simulink model "inversor"  (R2018a)
settings: Solver=VariableStepAuto  StartTime=0.0  StopTime=2  MaxStep=1e-4  RelTol=1e-3
InitFcn:
  | stateStadeInv
  | MODELOHIDROV8
undefined symbols (not defined in the file): Fr, sigbuilder_block
libraries: simulink x2, powerlib x1
settings Model: Creator=Hp 14  LastModifiedBy=cmparedes

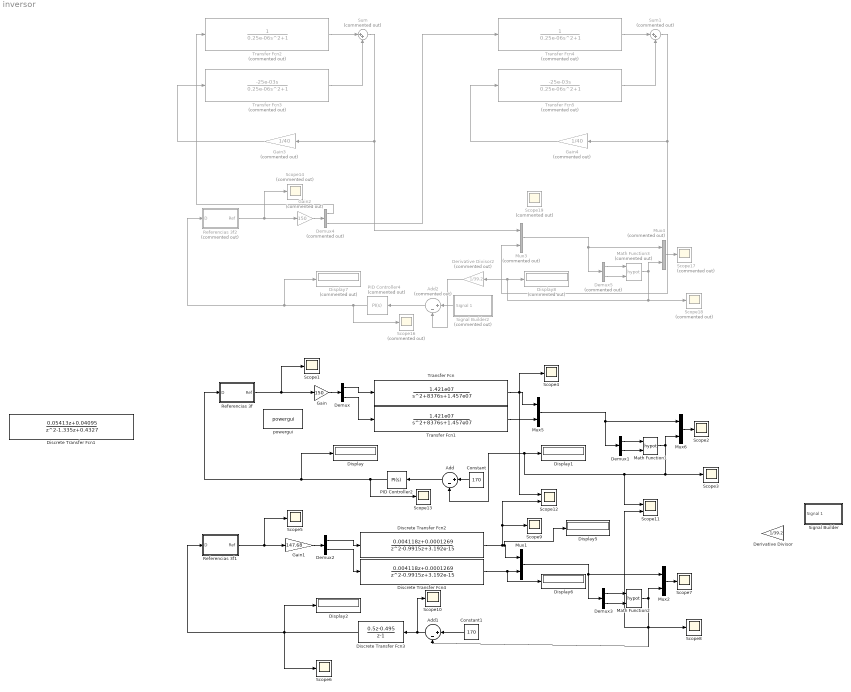
== system inversor ==
  Add : Sum  Inputs=|+-
  Add1 : Sum  Inputs=|+-
  Add2 : Sum  Commented=on  Inputs=|+-
  Constant : Constant  Value=170
  Constant1 : Constant  Value=170
  Demux{,1..3} (4 alike) : Demux  Outputs=2
  Demux4 : Demux  Commented=on  Outputs=2
  Demux5 : Demux  Commented=on  Outputs=2
  Derivative Divisor : Gain  Gain=1/39.2  SaturateOnIntegerOverflow=on  OutDataTypeStr=Inherit: Same as input  ParamDataTypeStr=Inherit: Same as input
  Derivative Divisor2 : Gain  Commented=on  Gain=1/39.2  SaturateOnIntegerOverflow=on  OutDataTypeStr=Inherit: Same as input  ParamDataTypeStr=Inherit: Same as input
  Discrete Transfer Fcn1 : DiscreteTransferFcn  Numerator=[0.05413 0.04095]  Denominator=[1 -1.335 0.4327]
  Discrete Transfer Fcn2 : DiscreteTransferFcn  Numerator=[0.004118 0.0001269]  Denominator=[1 -0.9915 3.192e-15]
  Discrete Transfer Fcn3 : DiscreteTransferFcn  Numerator=[0.5 -0.495]  Denominator=[1 -1]
  Discrete Transfer Fcn4 : DiscreteTransferFcn  Numerator=[0.004118 0.0001269]  Denominator=[1 -0.9915 3.192e-15]
  Display{,1..2,5..6} (5 alike) : Display
  Display7 : Display  Commented=on
  Display8 : Display  Commented=on
  Gain : Gain  Gain=150
  Gain1 : Gain  Gain=147.68
  Gain2 : Gain  Commented=on  Gain=150
  Gain3 : Gain  Commented=on  Gain=1/40
  Gain4 : Gain  Commented=on  Gain=1/40
  Math Function1 : Math  Operator=hypot  SaturateOnIntegerOverflow=on
  Math Function2 : Math  Operator=hypot  SaturateOnIntegerOverflow=on
  Math Function3 : Math  Commented=on  Operator=hypot  SaturateOnIntegerOverflow=on
  Mux{1..2,5..6} (4 alike) : Mux  Inputs=2
  Mux3 : Mux  Commented=on  Inputs=2
  Mux4 : Mux  Commented=on  Inputs=2
  PID Controller2 : simulink/Continuous/PID Controller  Controller=PI  TimeDomain=Continuous-time  SampleTime=-1  IntegratorMethod=Forward Euler  FilterMethod=Forward Euler  Form=Parallel  UseFilter=on  ControllerParametersSource=internal  P=0.5  I=50  D=0  N=100  InitialConditionSource=internal  InitialConditionForIntegrator=0  InitialConditionForFilter=0  ExternalReset=none  LimitOutput=off  UpperSaturationLimit=inf  LowerSaturationLimit=-inf  LinearizeAsGain=on  AntiWindupMode=none  Kb=1  TrackingMode=off  Kt=1  PParamMin=[]  PParamMax=[]  IParamMin=[]  IParamMax=[]  DParamMin=[]  DParamMax=[]  NParamMin=[]  NParamMax=[]  KbParamMin=[]  KbParamMax=[]  KtParamMin=[]  KtParamMax=[]  POutMin=[]  POutMax=[]  IOutMin=[]  IOutMax=[]  DOutMin=[]  DOutMax=[]  NOutMin=[]  NOutMax=[]  KbOutMin=[]  KbOutMax=[]  KtOutMin=[]  KtOutMax=[]  IntegratorOutMin=[]  IntegratorOutMax=[]  FilterOutMin=[]  FilterOutMax=[]  SumOutMin=[]  SumOutMax=[]  SumI1OutMin=[]  SumI1OutMax=[]  SumI2OutMin=[]  SumI2OutMax=[]  SumI3OutMin=[]  SumI3OutMax=[]  SumDOutMin=[]  SumDOutMax=[]  SaturationOutMin=[]  SaturationOutMax=[]  IntegratorContinuousStateAttributes=''  IntegratorStateMustResolveToSignalObject=off  IntegratorRTWStateStorageClass=Auto  FilterContinuousStateAttributes=''  FilterStateMustResolveToSignalObject=off  FilterRTWStateStorageClass=Auto  DifferentiatorICPrevScaledInput=0  DifferentiatorOutMin=[]  DifferentiatorOutMax=[]  InitialConditionSetting=State (most efficient)  FilterDiffOutCoefMin=[]  FilterDiffOutCoefMax=[]  SumDenOutMin=[]  SumDenOutMax=[]  SumNumOutMin=[]  SumNumOutMax=[]  ReciprocalOutMin=[]  ReciprocalOutMax=[]  DivideOutMin=[]  DivideOutMax=[]  TunerSelectOption=Transfer Function Based (PID Tuner App)
  PID Controller4 : simulink/Continuous/PID Controller  Commented=on  Controller=PI  TimeDomain=Continuous-time  SampleTime=-1  IntegratorMethod=Forward Euler  FilterMethod=Forward Euler  Form=Parallel  UseFilter=on  ControllerParametersSource=internal  P=0.5  I=50  D=0  N=100  InitialConditionSource=internal  InitialConditionForIntegrator=0  InitialConditionForFilter=0  ExternalReset=none  LimitOutput=off  UpperSaturationLimit=inf  LowerSaturationLimit=-inf  LinearizeAsGain=on  AntiWindupMode=none  Kb=1  TrackingMode=off  Kt=1  PParamMin=[]  PParamMax=[]  IParamMin=[]  IParamMax=[]  DParamMin=[]  DParamMax=[]  NParamMin=[]  NParamMax=[]  KbParamMin=[]  KbParamMax=[]  KtParamMin=[]  KtParamMax=[]  POutMin=[]  POutMax=[]  IOutMin=[]  IOutMax=[]  DOutMin=[]  DOutMax=[]  NOutMin=[]  NOutMax=[]  KbOutMin=[]  KbOutMax=[]  KtOutMin=[]  KtOutMax=[]  IntegratorOutMin=[]  IntegratorOutMax=[]  FilterOutMin=[]  FilterOutMax=[]  SumOutMin=[]  SumOutMax=[]  SumI1OutMin=[]  SumI1OutMax=[]  SumI2OutMin=[]  SumI2OutMax=[]  SumI3OutMin=[]  SumI3OutMax=[]  SumDOutMin=[]  SumDOutMax=[]  SaturationOutMin=[]  SaturationOutMax=[]  IntegratorContinuousStateAttributes=''  IntegratorStateMustResolveToSignalObject=off  IntegratorRTWStateStorageClass=Auto  FilterContinuousStateAttributes=''  FilterStateMustResolveToSignalObject=off  FilterRTWStateStorageClass=Auto  DifferentiatorICPrevScaledInput=0  DifferentiatorOutMin=[]  DifferentiatorOutMax=[]  InitialConditionSetting=State (most efficient)  FilterDiffOutCoefMin=[]  FilterDiffOutCoefMax=[]  SumDenOutMin=[]  SumDenOutMax=[]  SumNumOutMin=[]  SumNumOutMax=[]  ReciprocalOutMin=[]  ReciprocalOutMax=[]  DivideOutMin=[]  DivideOutMax=[]  TunerSelectOption=Transfer Function Based (PID Tuner App)
  Referencias 3f : Subsystem
  Referencias 3f1 : Subsystem
  Referencias 3f2 : Subsystem  Commented=on
  Scope{1..10,13} (11 alike) : Scope
  Scope11 : Scope  NumInputPorts=2
  Scope12 : Scope  NumInputPorts=2
  Scope{14,16..19} (5 alike) : Scope  Commented=on
  Signal Builder : Subsystem  Tag=STV Subsys  LoadFcn=sigbuilder_block('load');  StartFcn=sigbuilder_block('start');  StopFcn=sigbuilder_block('stop');  ClipboardFcn=sigbuilder_block('clipboard');  mask(Sigbuilder block){tuvar=[0:10]}
      mask help: Sigbuilder GUI
      mask init:
      | if ~strcmp(get_param(bdroot(gcbh),'SimulationStatus'),'stopped') tuvar = sigbuilder_block('maskInit'); end
      settings: CopyFcn=sigbuilder_block('copy');  DeleteFcn=sigbuilder_block('delete');  ModelCloseFcn=sigbuilder_block('modelClose');  PreSaveFcn=sigbuilder_block('preSave');  PauseFcn=sigbuilder_block('pause')  ContinueFcn=sigbuilder_block('continue')  NameChangeFcn=sigbuilder_block('namechange');  OpenFcn=sigbuilder_block('open',[6 24 765 492 ]);  CloseFcn=sigbuilder_block('close');
      mask Display: plot(0, 0, 100, 100,[2, 2, 32, 32, 2], [68, 8, 8, 68, 68],[32, 2], [38, 38], [32, 19, 2],[53, 60, 44], [32, 17, 17, 2],[16, 16, 31, 31]);txt = getActiveGroup(gcbh);text(2, 100, txt,'verticalAlignment', 'top');
  Signal Builder2 : Subsystem  Tag=STV Subsys  Commented=on  LoadFcn=sigbuilder_block('load');  StartFcn=sigbuilder_block('start');  StopFcn=sigbuilder_block('stop');  ClipboardFcn=sigbuilder_block('clipboard');  mask(Sigbuilder block){tuvar=[0:10]}
      mask help: Sigbuilder GUI
      mask init:
      | if ~strcmp(get_param(bdroot(gcbh),'SimulationStatus'),'stopped') tuvar = sigbuilder_block('maskInit'); end
      settings: CopyFcn=sigbuilder_block('copy');  DeleteFcn=sigbuilder_block('delete');  ModelCloseFcn=sigbuilder_block('modelClose');  PreSaveFcn=sigbuilder_block('preSave');  PauseFcn=sigbuilder_block('pause')  ContinueFcn=sigbuilder_block('continue')  NameChangeFcn=sigbuilder_block('namechange');  OpenFcn=sigbuilder_block('open',[6 24 765 492 ]);  CloseFcn=sigbuilder_block('close');
      mask Display: plot(0, 0, 100, 100,[2, 2, 32, 32, 2], [68, 8, 8, 68, 68],[32, 2], [38, 38], [32, 19, 2],[53, 60, 44], [32, 17, 17, 2],[16, 16, 31, 31]);txt = getActiveGroup(gcbh);text(2, 100, txt,'verticalAlignment', 'top');
  Sum : Sum  Commented=on  Inputs=|++
  Sum1 : Sum  Commented=on  Inputs=|++
  Transfer Fcn : TransferFcn  Numerator=[1.421e07]  Denominator=[1 8376 1.457e07]
  Transfer Fcn1 : TransferFcn  Numerator=[1.421e07]  Denominator=[1 8376 1.457e07]
  Transfer Fcn2 : TransferFcn  Commented=on  Denominator=[0.25e-06 0 1]
  Transfer Fcn3 : TransferFcn  Commented=on  Numerator=[-25e-03 0]  Denominator=[0.25e-06 0 1]
  Transfer Fcn4 : TransferFcn  Commented=on  Denominator=[0.25e-06 0 1]
  Transfer Fcn5 : TransferFcn  Commented=on  Numerator=[-25e-03 0]  Denominator=[0.25e-06 0 1]
  powergui : powerlib/powergui  Priority=1  SimulationMode=Continuous  SampleTime=50e-3  frequency=60  Iterations=50  frequencyindice=0  Pbase=100e6  ErrMax=1e-4  UnitsV=kV  UnitsW=MW  buscounter=0  FunctionMessages=off  echomessages=off  EnableUseOfTLC=off  CurrentSourceSwitches=off  DisableSnubberDevices=off  DisableRonSwitches=off  DisableVfSwitches=off  DisplayEquations=off  SolverType=Tustin/Backward Euler (TBE)  Interpol=off  ExternalGateDelay=off  methode=off  Ts=100  x0status=blocks  SPID=on  SwTol=0  HookPort=off  RestoreLinks=warning  ResistiveCurrentMeasurement=off  Frange=[0:2:500]  Ylog=off  Xlog=on  ShowGrid=off  save=off  variable=ZData  structure=0  ZoomFFT=off  StartTime=0.0  cycles=1  DisplayStyle=1  fundamental=60  FreqAxis=off  MaxFrequency=1000  frequencyindicesteady=0 Hz  RmsSteady=1  display=off
  wires:
  Transfer Fcn1/1 -> Mux5/2
  Transfer Fcn/1 -> Scope12/1, Scope4/1, Mux5/1
  Demux1/1 -> Math Function1/1
  Mux5/1 -> Demux1/1, Mux6/1
  Mux6/1 -> Scope2/1
  Demux1/2 -> Math Function1/2
  Referencias 3f/1(Ref) -> Gain/1, Scope1/1
  Demux/1 -> Transfer Fcn/1
  Demux/2 -> Transfer Fcn1/1
  Gain/1 -> Demux/1
  PID Controller2/1 -> Display/1, Referencias 3f/1(D), Scope13/1
  Constant/1 -> Add/1
  Add/1 -> PID Controller2/1
  Math Function1/1 -> Mux6/2, Scope3/1, Add/2, Display1/1, Scope11/1
  Add1/1 -> Discrete Transfer Fcn3/1, Scope10/1
  Math Function2/1 -> Add1/2, Scope11/2, Scope8/1, Mux2/2
  Discrete Transfer Fcn3/1 -> Scope6/1, Referencias 3f1/1(D), Display2/1
  Referencias 3f1/1(Ref) -> Scope5/1, Gain1/1
  Demux3/2 -> Math Function2/2
  Mux2/1 -> Scope7/1
  Mux1/1 -> Mux2/1, Demux3/1
  Demux3/1 -> Math Function2/1
  Discrete Transfer Fcn2/1 -> Display5/1, Mux1/1, Scope12/2, Scope9/1
  Discrete Transfer Fcn4/1 -> Display6/1, Mux1/2
  Gain1/1 -> Demux2/1
  Demux2/1 -> Discrete Transfer Fcn2/1
  Demux2/2 -> Discrete Transfer Fcn4/1
  Derivative Divisor2/1 -> Add2/2
  Add2/1 -> PID Controller4/1
  Math Function3/1 -> Display8/1, Derivative Divisor2/1, Scope18/1, Mux4/2
  Signal Builder2/1(Signal 1) -> Add2/1
  PID Controller4/1 -> Scope16/1, Referencias 3f2/1(D), Display7/1
  Gain2/1 -> Demux4/1
  Referencias 3f2/1(Ref) -> Scope14/1, Gain2/1
  Demux5/2 -> Math Function3/2
  Mux4/1 -> Scope17/1
  Mux3/1 -> Mux4/1, Demux5/1
  Demux5/1 -> Math Function3/1
  Demux4/1 -> Transfer Fcn2/1
  Gain3/1 -> Transfer Fcn3/1
  Transfer Fcn2/1 -> Sum/1
  Sum/1 -> Mux3/1, Gain3/1
  Transfer Fcn3/1 -> Sum/2
  Transfer Fcn5/1 -> Sum1/2
  Sum1/1 -> Mux3/2, Gain4/1
  Transfer Fcn4/1 -> Sum1/1
  Gain4/1 -> Transfer Fcn5/1
  Demux4/2 -> Transfer Fcn4/1
  Constant1/1 -> Add1/1

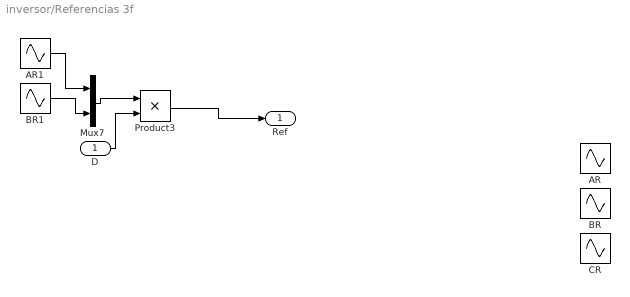
== system inversor/Referencias 3f ==
  D : Inport
  AR : Sin  Frequency=Fr*2*pi  SampleTime=0
  AR1 : Sin  Frequency=Fr*2*pi  SampleTime=0
  BR : Sin  Frequency=Fr*2*pi  Phase=-2*pi/3  SampleTime=0
  BR1 : Sin  Frequency=Fr*2*pi  Phase=-pi/2  SampleTime=0
  CR : Sin  Frequency=Fr*2*pi  Phase=2*pi/3  SampleTime=0
  Mux7 : Mux  Inputs=2
  Product3 : Product  OutDataTypeStr=double  RndMeth=Zero
  Ref : Outport
  wires:
  BR1/1 -> Mux7/2
  AR1/1 -> Mux7/1
  Mux7/1 -> Product3/1
  D/1 -> Product3/2
  Product3/1 -> Ref/1

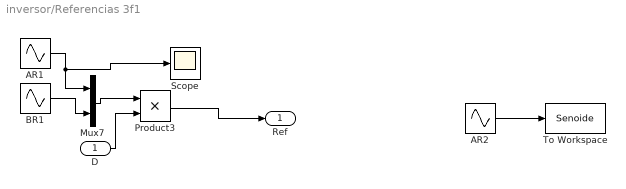
== system inversor/Referencias 3f1 ==
  D : Inport
  AR1 : Sin  Frequency=Fr*2*pi  SampleTime=0
  AR2 : Sin  Frequency=Fr*2*pi  SampleTime=0
  BR1 : Sin  Frequency=Fr*2*pi  Phase=-pi/2  SampleTime=0
  Mux7 : Mux  Inputs=2
  Product3 : Product  OutDataTypeStr=double  RndMeth=Zero
  Scope : Scope
  To Workspace : ToWorkspace  VariableName=Senoide  SaveFormat=Timeseries  SampleTime=-1
  Ref : Outport
  wires:
  Product3/1 -> Ref/1
  D/1 -> Product3/2
  Mux7/1 -> Product3/1
  AR1/1 -> Scope/1, Mux7/1
  BR1/1 -> Mux7/2
  AR2/1 -> To Workspace/1

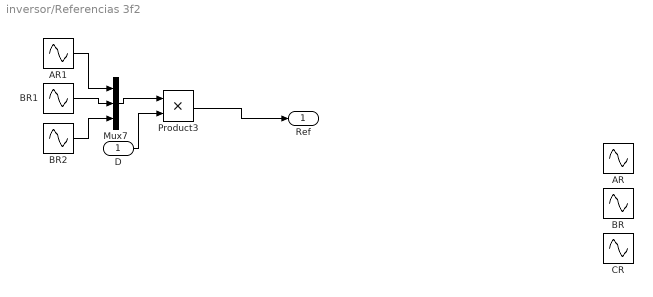
== system inversor/Referencias 3f2 ==
  D : Inport
  AR : Sin  Frequency=Fr*2*pi  SampleTime=0
  AR1 : Sin  Frequency=Fr*2*pi  SampleTime=0
  BR : Sin  Frequency=Fr*2*pi  Phase=-2*pi/3  SampleTime=0
  BR1 : Sin  Frequency=Fr*2*pi  Phase=-pi/2  SampleTime=0
  BR2 : Sin  Frequency=Fr*2*pi  Phase=pi/2  SampleTime=0
  CR : Sin  Frequency=Fr*2*pi  Phase=2*pi/3  SampleTime=0
  Mux7 : Mux  Inputs=3
  Product3 : Product  OutDataTypeStr=double  RndMeth=Zero
  Ref : Outport
  wires:
  Product3/1 -> Ref/1
  D/1 -> Product3/2
  Mux7/1 -> Product3/1
  AR1/1 -> Mux7/1
  BR1/1 -> Mux7/2
  BR2/1 -> Mux7/3

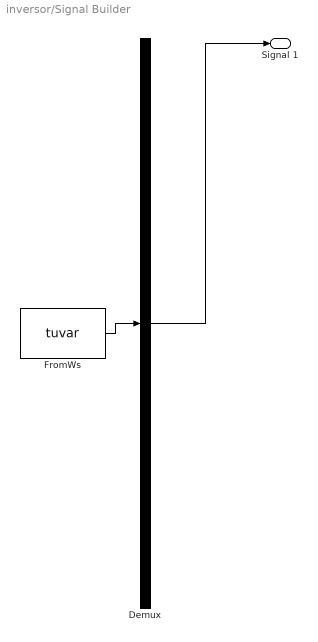
== system inversor/Signal Builder ==
  Demux : Demux  Tag=STV Demux  Outputs=1
  FromWs : FromWorkspace  Tag=STV FromWs  VariableName=tuvar  SampleTime=0
      SigBuilderData=|
      | common.afterFinalStr = 'Extrapolate'
      | common.sampleTime = 0
      | dataSet.timeRange = [0 1]
      | dataSet.name = 'Group 1'
      | sbobj.Name = 'Signal Builder'
      | sbobj.Groups.Name = 'Group 1'
      | sbobj.Groups.Signals.Name = 'Signal 1'
      | sbobj.Groups.Signals.XData = [0 1]
      | sbobj.Groups.Signals.YData = [1 1]
      | sbobj.Groups.TimeRange = [0 1]
  Signal 1 : Outport  Tag=STV Outport
  wires:
  FromWs/1 -> Demux/1
  Demux/1 -> Signal 1/1

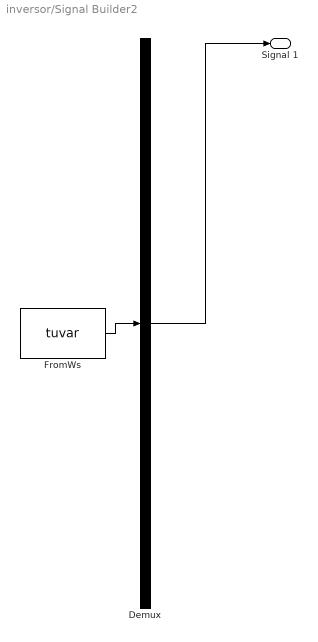
== system inversor/Signal Builder2 ==
  Demux : Demux  Tag=STV Demux  Outputs=1
  FromWs : FromWorkspace  Tag=STV FromWs  VariableName=tuvar  SampleTime=0
      SigBuilderData=|
      | common.afterFinalStr = 'Extrapolate'
      | common.sampleTime = 0
      | dataSet.timeRange = [0 1]
      | dataSet.name = 'Group 1'
      | sbobj.Name = 'Signal Builder'
      | sbobj.Groups.Name = 'Group 1'
      | sbobj.Groups.Signals.Name = 'Signal 1'
      | sbobj.Groups.Signals.XData = [0 1]
      | sbobj.Groups.Signals.YData = [1 1]
      | sbobj.Groups.TimeRange = [0 1]
  Signal 1 : Outport  Tag=STV Outport
  wires:
  Demux/1 -> Signal 1/1
  FromWs/1 -> Demux/1
